simulink model "EV_thermal_charger_2015a_jmaab"  (R2015a)
settings: Solver=ode3  StartTime=0.0  StopTime=1800  FixedStep=sampling_time  RelTol=1e-3
PreLoadFcn:
  | run('init_setting.m')
PostLoadFcn:
  | %set_param(gcs, 'SimulationCommand', 'update');
  | %load('save_param/save_P_Charger', 'P_Charger');
  | %load('save_param/save_T_User_set_temp_degC','T_User_set_temp_degC');
  | %load('save_param/save_ENV_PNT_PTTH_Temp_add_degC','ENV_PNT_PTTH_Temp_add_degC');
  | %load('save_param/save_ENV_PNT_CABIN_Temp_add_degC','ENV_PNT_CABIN_Temp_add_degC');
  | %load('save_param/save_ENV_PNT_PHI_Sunlight_W','ENV_PNT_PHI_Sunlight_W');
  | %load('save_param/save_ENV_PNT_Outside_Temp_ini_degC','ENV_PNT_Outside_Temp_ini_degC');
undefined symbols (not defined in the file or in its folder): BK_PNT_Pow_UL, BK_PNT_ReGene_vel_limit_DN_kmph, BK_PNT_ReGene_vel_limit_UP_kmph, BK_PNT_Tau_brake, Brk_LL, Brk_PGain, Brk_UL, BT_PNT_Hi_C_pol_hi_batt, BT_PNT_Hi_Capa_hi_batt_F, BT_PNT_Hi_ocv_SOC_hi_batt_OCV_V_table, BT_PNT_Hi_ocv_SOC_hi_batt_OCV_V_table_x_SOC, BT_PNT_Hi_R_hi_batt_cell, BT_PNT_Hi_R_pol_hi_batt, BT_PNT_Hi_SOC_MAX_hi_batt, BT_PNT_Hi_SOC_MIN_hi_batt, BT_PNT_Hi_SOC_START_hi_batt, BT_PNT_Lo_Capa_lo_batt_F, BT_PNT_Lo_ocv_SOC_lo_batt_OCV_V_table, BT_PNT_Lo_ocv_SOC_lo_batt_OCV_V_table_x_SOC, BT_PNT_Lo_R_lo_batt_ohm, BT_PNT_Lo_SOC_MAX_lo_batt, BT_PNT_Lo_SOC_MIN_lo_batt, BT_PNT_Lo_SOC_START_lo_batt, BTTH_CNT_P_BT_Heater_W, BTTH_CNT_P_BT_Heater_W_x_BTCells_degC, BTTH_CNT_Voltage_BTFan_V, BTTH_CNT_Voltage_BTFan_V_x_BTCells_degC, BTTH_PNT_BT_Heat_Resi_KpW, BTTH_PNT_BT_Heat_Resi_KpW_x_Wind_m3ps, BTTH_PNT_BT_Heater2BTCells_Heat_Resi_KpW, BTTH_PNT_BT_Heater_Heat_Capa_JpK, BTTH_PNT_BTBlock2BTAir_Heat_Resi_KpW, BTTH_PNT_BTBlock_Heat_Capa_JpK, BTTH_PNT_BTCells2BTBlock_Heat_Resi_KpW, BTTH_PNT_BTCells_Heat_Capa_JpK, BTTH_PNT_v_BTFan_Wind_vel_mps, BTTH_PNT_v_BTFan_Wind_vel_mps_x_V_BTFan, CATH_CNT_P_Aircon_W_LL, CATH_CNT_P_Aircon_W_UL, CATH_CNT_P_Gain_Aircon, CATH_CNT_P_Gain_PTC_Heater, CATH_CNT_P_Gain_SeatHT, CATH_CNT_P_PTC_Heater, CATH_CNT_P_PTC_Heater_W_LL, CATH_CNT_P_PTC_Heater_W_UL, CATH_CNT_P_PTC_Heater_x_T_Outside_temp_degC, CATH_CNT_P_SeatHT_W_LL, CATH_CNT_P_SeatHT_W_UL, CATH_CNT_PGain_Temp_blowout, CATH_CNT_T_Aircon_Indoor_degC, CATH_CNT_T_Aircon_Indoor_degC_x_T_blowout_degC, CATH_CNT_T_PTC_Heater_degC_UL, CATH_CNT_T_SeatHT_Temp_degC, CATH_CNT_T_SeatHT_Temp_degC_x_T_blowout_degC, CATH_CNT_V_HVAC_Fan, CATH_CNT_V_HVAC_Fan_x_T_blowout_degC, CATH_CNT_V_RDFan_V, CATH_CNT_V_RDFan_x_P_Aircon_W, CATH_PNT_Air_Convection_Heat_Resi_KpW, CATH_PNT_Air_Convection_Heat_Resi_x_mps ... (+142)
undefined symbols (not defined in the file): ACC_D_Gain, ACC_I_Gain, ACC_P_Gain
libraries: METI_Lib_vehicle_model x52, simulink x35
(part 3 of 6)

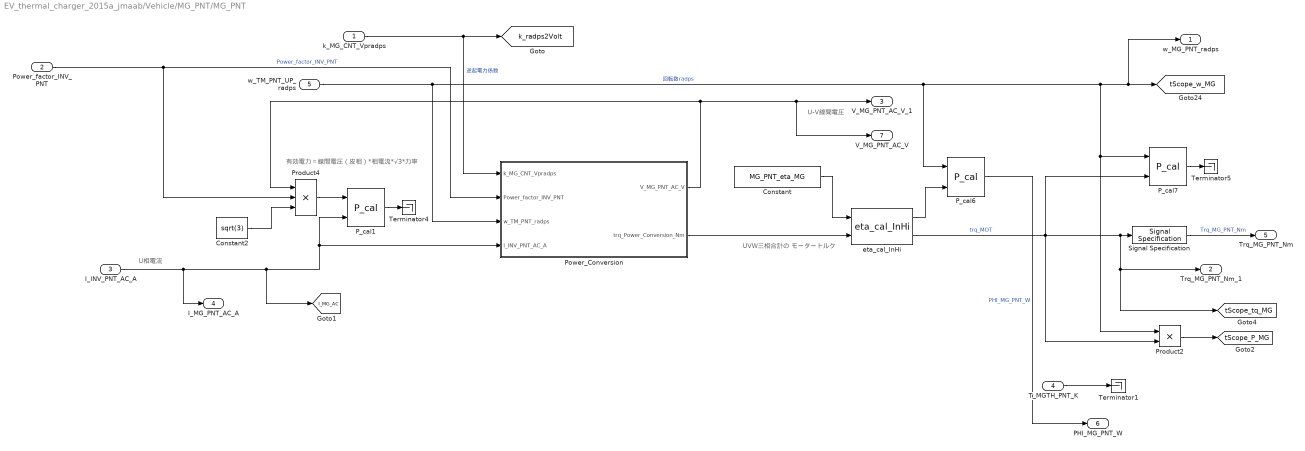
== system EV_thermal_charger_2015a_jmaab/Vehicle/MG_PNT/MG_PNT ==
  note: UVW三相合計の
      | モータートルク
  note: U-V線間電圧
  note: U相電流
  note: 有効電力＝線間電圧（皮相）*相電流*√3*力率
  k_MG_CNT_Vpradps : Inport
  Power_factor_INV_PNT : Inport  Port=2
  "I_INV_PNT_AC_A " : Inport  Port=3
  T_MGTH_PNT_K : Inport  Port=4
  w_TM_PNT_UP_radps : Inport  Port=5
  Constant : Constant  Value=MG_PNT_eta_MG
  Constant2 : Constant  Value=sqrt(3)
  P_cal1 : METI_Lib_vehicle_model/P_cal  Type_energy=電気  Type_output_energy=出力  Power_name=Po_  t_Workspace_Name=MG_PNT_ELEC  P_VariableName=Po_MG_PNT_ELEC  Across_VariableName=V_MG_PNT_ELEC  Throgh_VariableName=I_MG_PNT_ELEC
  P_cal6 : METI_Lib_vehicle_model/P_cal  Type_energy=回転運動  Type_output_energy=損失  Power_name=Pl_  t_Workspace_Name=MG_PNT_FRIC_LOSS  P_VariableName=Pl_MG_PNT_FRIC_LOSS  Across_VariableName=w_MG_PNT_FRIC_LOSS  Throgh_VariableName=tq_MG_PNT_FRIC_LOSS
  P_cal7 : METI_Lib_vehicle_model/P_cal  Type_energy=回転運動  Type_output_energy=出力  Power_name=Po_  t_Workspace_Name=MG_PNT_ROT  P_VariableName=Po_MG_PNT_ROT  Across_VariableName=w_MG_PNT_ROT  Throgh_VariableName=tq_MG_PNT_ROT
  Power_Conversion : Subsystem
  Product2 : Product
  Product4 : Product  Inputs=3
  Signal Specification : SignalSpecification
  Terminator1 : Terminator
  Terminator4 : Terminator
  Terminator5 : Terminator
  eta_cal_InHi : METI_Lib_vehicle_model/eta_cal_InHi  SystemSampleTime=-1
  w_MG_PNT_radps : Outport
  "Trq_MG_PNT_Nm_1 " : Outport  Port=2
  V_MG_PNT_AC_V_1 : Outport  Port=3
  I_MG_PNT_AC_A : Outport  Port=4
  Trq_MG_PNT_Nm : Outport  Port=5
  "PHI_MG_PNT_W " : Outport  Port=6
  "V_MG_PNT_AC_V " : Outport  Port=7
  tag scope: I_MG_AC=global, k_radps2Volt=global, tScope_P_MG=global, tScope_tq_MG=global, tScope_w_MG=global
  wires:
  P_cal1/1 -> Terminator4/1
  P_cal7/1 -> Terminator5/1
  w_TM_PNT_UP_radps/1 -> Power_Conversion/3("w_TM_PNT_radps "), w_MG_PNT_radps/1, [tScope_w_MG], Product2/1, P_cal7/1, P_cal6/1  "回転数radps"
  eta_cal_InHi/2 -> P_cal7/2, Product2/2, [tScope_tq_MG], "Trq_MG_PNT_Nm_1 "/1, Signal Specification/1  "trq_MOT"
  Product2/1 -> [tScope_P_MG]
  P_cal6/1 -> "PHI_MG_PNT_W "/1  "PHI_MG_PNT_W"
  Constant/1 -> eta_cal_InHi/1
  eta_cal_InHi/1 -> P_cal6/2
  k_MG_CNT_Vpradps/1 -> [k_radps2Volt], Power_Conversion/1(k_MG_CNT_Vpradps)  "逆起電力係数"
  Power_Conversion/2("trq_Power_Conversion_Nm ") -> eta_cal_InHi/2
  Power_Conversion/1(V_MG_PNT_AC_V) -> Product4/1, V_MG_PNT_AC_V_1/1, "V_MG_PNT_AC_V "/1
  Product4/1 -> P_cal1/1
  "I_INV_PNT_AC_A "/1 -> [I_MG_AC], P_cal1/2, Power_Conversion/4("I_INV_PNT_AC_A "), I_MG_PNT_AC_A/1
  Power_factor_INV_PNT/1 -> Power_Conversion/2(Power_factor_INV_PNT), Product4/2  "Power_factor_INV_PNT"
  Constant2/1 -> Product4/3
  T_MGTH_PNT_K/1 -> Terminator1/1
  Signal Specification/1 -> Trq_MG_PNT_Nm/1  "Trq_MG_PNT_Nm"

== system EV_thermal_charger_2015a_jmaab/Vehicle/VL_PNT/cal_Hill_Climbing_Resi ==
  note: 登坂抵抗
  In1 : Inport
  Constant2 : Constant  Value=g
  Constant3 : Constant  Value=M
  Gain : Gain  Gain=deg2rad
  Product1 : Product
  Product3 : Product
  Trigonometric Function : Trigonometry
  Out1 : Outport
  wires:
  Trigonometric Function/1 -> Product1/2
  Product1/1 -> Out1/1
  Product3/1 -> Product1/1
  Gain/1 -> Trigonometric Function/1
  Constant2/1 -> Product3/2
  Constant3/1 -> Product3/1
  In1/1 -> Gain/1

== system EV_thermal_charger_2015a_jmaab/Driver/Caliculate_Opeining_Accel/FB/Filter ==
  In1 : Inport
  Gain3 : Gain  Gain=10
  Gain4 : Gain  Gain=0.1
  Rounding Function : Rounding  Operator=round
  Out1 : Outport
  wires:
  Rounding Function/1 -> Gain4/1
  In1/1 -> Gain3/1
  Gain3/1 -> Rounding Function/1
  Gain4/1 -> Out1/1

== system EV_thermal_charger_2015a_jmaab/Driver/Caliculate_Opeining_Accel/FF1/Subsystem ==
  Req_Force : Inport
  Upper_Acc_Force_Input : Inport  Port=2
  Upper_ACC_percent : Inport  Port=3
  Lower_Acc_Force_Input : Inport  Port=4
  Lower_Acc_percent : Inport  Port=5
  Add10 : Sum
  Add11 : Sum  Inputs=+-
  Add8 : Sum  Inputs=+-
  Add9 : Sum  Inputs=+-
  Compare To Zero1 : simulink/Logic and Bit Operations/Compare To Zero  relop=>  OutDataTypeStr=boolean
  Divide_0wari2 : METI_Lib_vehicle_model/Divide_0wari
  Product2 : Product
  Acc_percent_Out : Outport
  threshold_Out : Outport  Port=2
  wires:
  Compare To Zero1/1 -> threshold_Out/1
  Req_Force/1 -> Add9/1
  Lower_Acc_Force_Input/1 -> Add9/2, Add8/2
  Add11/1 -> Product2/2
  Lower_Acc_percent/1 -> Add10/2, Add11/2
  Upper_Acc_Force_Input/1 -> Add8/1
  Product2/1 -> Add10/1
  Add8/1 -> Divide_0wari2/2
  Divide_0wari2/1 -> Product2/1
  Add9/1 -> Compare To Zero1/1, Divide_0wari2/1
  Upper_ACC_percent/1 -> Add11/1
  Add10/1 -> Acc_percent_Out/1

== system EV_thermal_charger_2015a_jmaab/Driver/Caliculate_Opeining_Accel/FF1/Subsystem1 ==
  Req_Force : Inport
  Upper_Acc_Force_Input : Inport  Port=2
  Upper_ACC_percent : Inport  Port=3
  Lower_Acc_Force_Input : Inport  Port=4
  Lower_Acc_percent : Inport  Port=5
  Add10 : Sum
  Add11 : Sum  Inputs=+-
  Add8 : Sum  Inputs=+-
  Add9 : Sum  Inputs=+-
  Compare To Zero1 : simulink/Logic and Bit Operations/Compare To Zero  relop=>  OutDataTypeStr=boolean
  Divide_0wari2 : METI_Lib_vehicle_model/Divide_0wari
  Product2 : Product
  Acc_percent_Out : Outport
  threshold_Out : Outport  Port=2
  wires:
  Compare To Zero1/1 -> threshold_Out/1
  Req_Force/1 -> Add9/1
  Lower_Acc_Force_Input/1 -> Add9/2, Add8/2
  Add11/1 -> Product2/2
  Lower_Acc_percent/1 -> Add10/2, Add11/2
  Upper_Acc_Force_Input/1 -> Add8/1
  Product2/1 -> Add10/1
  Add8/1 -> Divide_0wari2/2
  Divide_0wari2/1 -> Product2/1
  Add9/1 -> Compare To Zero1/1, Divide_0wari2/1
  Upper_ACC_percent/1 -> Add11/1
  Add10/1 -> Acc_percent_Out/1

== system EV_thermal_charger_2015a_jmaab/Driver/Caliculate_Opeining_Accel/FF1/Subsystem2 ==
  Req_Force : Inport
  Upper_Acc_Force_Input : Inport  Port=2
  Upper_ACC_percent : Inport  Port=3
  Lower_Acc_Force_Input : Inport  Port=4
  Lower_Acc_percent : Inport  Port=5
  Add10 : Sum
  Add11 : Sum  Inputs=+-
  Add8 : Sum  Inputs=+-
  Add9 : Sum  Inputs=+-
  Compare To Zero1 : simulink/Logic and Bit Operations/Compare To Zero  relop=>  OutDataTypeStr=boolean
  Divide_0wari2 : METI_Lib_vehicle_model/Divide_0wari
  Product2 : Product
  Acc_percent_Out : Outport
  threshold_Out : Outport  Port=2
  wires:
  Compare To Zero1/1 -> threshold_Out/1
  Req_Force/1 -> Add9/1
  Lower_Acc_Force_Input/1 -> Add9/2, Add8/2
  Add11/1 -> Product2/2
  Lower_Acc_percent/1 -> Add10/2, Add11/2
  Upper_Acc_Force_Input/1 -> Add8/1
  Product2/1 -> Add10/1
  Add8/1 -> Divide_0wari2/2
  Divide_0wari2/1 -> Product2/1
  Add9/1 -> Compare To Zero1/1, Divide_0wari2/1
  Upper_ACC_percent/1 -> Add11/1
  Add10/1 -> Acc_percent_Out/1

== system EV_thermal_charger_2015a_jmaab/Driver/Caliculate_Opeining_Accel/FF1/慣性 ==
  v_tgt : Inport
  Add : Sum
  Constant : Constant  Value=M
  Constant1 : Constant  Value=1/2
  Derivative : Derivative
  Derivative1 : Derivative
  Divide1 : Product  Inputs=***
  Memory : Memory
  F_Inertia : Outport
  wires:
  Divide1/1 -> F_Inertia/1
  v_tgt/1 -> Derivative/1, Memory/1
  Add/1 -> Divide1/2
  Derivative/1 -> Add/1
  Derivative1/1 -> Add/2
  Memory/1 -> Derivative1/1
  Constant1/1 -> Divide1/1
  Constant/1 -> Divide1/3

== system EV_thermal_charger_2015a_jmaab/Driver/Caliculate_Opeining_Accel/FF1/空気抵抗 ==
  v_tgt : Inport
  V_wind : Constant  Value=0
  cal_Air_resi1 : METI_Lib_vehicle_model/vehicle_model/cal_Air_resi  Vel_max=200
  F_air_resi : Outport
  wires:
  cal_Air_resi1/1 -> F_air_resi/1
  V_wind/1 -> cal_Air_resi1/2
  v_tgt/1 -> cal_Air_resi1/1

== system EV_thermal_charger_2015a_jmaab/Driver/Caliculate_Opeining_Accel/FF1/転がり抵抗 ==
  v_tgt : Inport
  cal_roll_resi : METI_Lib_vehicle_model/vehicle_model/cal_roll_resi  Myu_tire=myu  Vehicle_Mass=M  Gravi_acc=g
  F_rollresi : Outport
  wires:
  cal_roll_resi/1 -> F_rollresi/1
  v_tgt/1 -> cal_roll_resi/1

== system EV_thermal_charger_2015a_jmaab/Vehicle/BAT_Hi_PNT/BT_Hi_PNT/Cal_SOC ==
  I_BT_PNT_A : Inport
  Capa_batt : Inport  Port=2
  SOC_st : Inport  Port=3
  SOC_MAX : Inport  Port=4
  SOC_MIN : Inport  Port=5
  Clock : Clock
  Memory : Memory
  Memory1 : Memory
  Saturation Dynamic : simulink/Discontinuities/Saturation Dynamic  OutMin=[]  OutMax=[]  OutDataTypeStr=Inherit: Same as second input  OutDataType=fixdt(1, 16)  OutScaling=2^-10  DoSatur=off
  Subsystem4 : Subsystem  mask{SOC=SOC_LoBat, VariableName=Asec_LoBat}
      mask prompts: SOC "バッテリSOC"; VariableName "バッテリ容量変化量(Asec)"
  Sum : Sum  Inputs=|++
  Sum1 : Sum  Inputs=++|
  Sum2 : Sum  Inputs=+-|
  Sum5 : Sum  Inputs=|+-
  capa_mn : Product  RndMeth=Zero
  capa_mx : Product  RndMeth=Zero
  capa_mx1 : Product  RndMeth=Zero
  capa_st : Product  RndMeth=Zero
  capa_st1 : Product  Inputs=*/  RndMeth=Zero
  h2sec : Gain  Gain=h2sec
  k : Gain  Gain=percent2mujigen
  k1 : Gain  Gain=percent2mujigen
  k2 : Gain  Gain=percent2mujigen
  k3 : Gain  Gain=mujigen2percent
  SOC_out : Outport
  wires:
  Sum5/1 -> capa_mx1/2
  Memory1/1 -> Sum5/2
  Sum/1 -> Saturation Dynamic/2
  Clock/1 -> Sum5/1, Memory1/1
  capa_mx1/1 -> Sum1/1
  k3/1 -> Subsystem4/1(In1), SOC_out/1
  Sum1/1 -> Sum/2
  Memory/1 -> Sum1/2
  k2/1 -> capa_st/2
  k1/1 -> capa_mn/2
  k/1 -> capa_mx/2
  capa_st/1 -> Sum2/2, Sum/1
  Saturation Dynamic/1 -> Sum2/1, capa_st1/1
  capa_mx/1 -> Saturation Dynamic/1
  capa_mn/1 -> Saturation Dynamic/3
  capa_st1/1 -> k3/1
  h2sec/1 -> capa_mn/1, capa_st1/2, capa_st/1, capa_mx/1
  SOC_MIN/1 -> k1/1
  SOC_MAX/1 -> k/1
  SOC_st/1 -> k2/1
  Capa_batt/1 -> h2sec/1
  I_BT_PNT_A/1 -> capa_mx1/1
  Sum2/1 -> Memory/1, Subsystem4/2(In2)

== system EV_thermal_charger_2015a_jmaab/Vehicle/BAT_Hi_PNT/BT_Hi_PNT/Subsystem ==
  I_BT_PNT_A : Inport
  Add : Sum
  Divide : Product
  Resistivity : Constant  Value=BT_PNT_Hi_R_hi_batt_cell
  Transfer Fcn : TransferFcn  Numerator=[BT_PNT_Hi_R_pol_hi_batt]  Denominator=[BT_PNT_Hi_R_pol_hi_batt*BT_PNT_Hi_C_pol_hi_batt 1]
  V_BT_PNT_V : Outport
  wires:
  Resistivity/1 -> Divide/2
  I_BT_PNT_A/1 -> Transfer Fcn/1, Divide/1
  Divide/1 -> Add/1
  Transfer Fcn/1 -> Add/2
  Add/1 -> V_BT_PNT_V/1

== system EV_thermal_charger_2015a_jmaab/Vehicle/BTTH/BTTH_PNT/BB_PNT ==
  note: バッテリ筐体の
      | 熱容量
  ini_T_Environment_Outside_degC : Inport
  T_ATM_PNT_BB_K : Inport  Port=2
  PHI_BTBlock1_W : Inport  Port=3
  BTBlock_Heat_Capacity : Subsystem
  BT_Block2Air_Heat_Resistance : Subsystem
  T_BTBlock1_K : Outport
  PHI_BB_PNT_ATM_W : Outport  Port=2
  T_BTBlock2_K : Outport  Port=3
  wires:
  ini_T_Environment_Outside_degC/1 -> BTBlock_Heat_Capacity/1(ini_T_Environment_Outside_degC)
  BTBlock_Heat_Capacity/1(T_BTBlock1_K) -> T_BTBlock1_K/1
  PHI_BTBlock1_W/1 -> BTBlock_Heat_Capacity/2(PHI_BTBlock1_W)
  BT_Block2Air_Heat_Resistance/1(PHI_BT2AIR_Resi1_W) -> PHI_BB_PNT_ATM_W/1  "PHI_BB_PNT_ATM_W"
  BT_Block2Air_Heat_Resistance/2(PHI_BTBlock_Resi2_W) -> BTBlock_Heat_Capacity/3(PHI_BTBlock2_W)
  T_ATM_PNT_BB_K/1 -> BT_Block2Air_Heat_Resistance/1(T_ATM_PNT_BB_K)
  BTBlock_Heat_Capacity/2(T_BTBlock2_K) -> T_BTBlock2_K/1, BT_Block2Air_Heat_Resistance/2(T_BTBlock_Resi2_K)

== system EV_thermal_charger_2015a_jmaab/Vehicle/BTTH/BTTH_PNT/BC_PNT ==
  note: バッテリセルの
      | 熱容量
  PHI_BTCells4_W : Inport
  T_BTBlock_Resi1_K : Inport  Port=2
  ini_T_Environment_Outside_degC : Inport  Port=3
  PHI_BTCells2_W : Inport  Port=4
  PHI_BT_HI_PNT_W : Inport  Port=5
  BTCells_Heat_Capacity : Subsystem
  BT_Cells2BTBlock_Heat_Resistance : Subsystem
  T_BTCells4_K : Outport
  PHI_BTBlock_Resi1_W : Outport  Port=2
  T_BC_PNT_K : Outport  Port=3
  T_BTCCell_K : Outport  Port=4
  T_BTCells2_K : Outport  Port=5
  wires:
  BTCells_Heat_Capacity/2(T_BTCells2_K) -> T_BTCells2_K/1
  PHI_BTCells2_W/1 -> BTCells_Heat_Capacity/3(PHI_BTCells2_W)
  ini_T_Environment_Outside_degC/1 -> BTCells_Heat_Capacity/1(ini_T_Environment_Outside_degC)
  PHI_BT_HI_PNT_W/1 -> BTCells_Heat_Capacity/2(PHI_BTCells1_W)
  PHI_BTCells4_W/1 -> BTCells_Heat_Capacity/5(PHI_BTCells4_W)
  BT_Cells2BTBlock_Heat_Resistance/2(PHI_BTCells_Resi2_W) -> BTCells_Heat_Capacity/4(PHI_BTCells3_W)
  BT_Cells2BTBlock_Heat_Resistance/1(PHI_BTBlock_Resi1_W) -> PHI_BTBlock_Resi1_W/1
  BTCells_Heat_Capacity/1(T_BTCells1_K) -> T_BC_PNT_K/1  "T_BC_PNT_K"
  T_BTBlock_Resi1_K/1 -> BT_Cells2BTBlock_Heat_Resistance/1(T_BTBlock_Resi1_K)
  BTCells_Heat_Capacity/4(T_BTCells4_K) -> T_BTCells4_K/1
  BTCells_Heat_Capacity/3(T_BTCells3_K) -> T_BTCCell_K/1, BT_Cells2BTBlock_Heat_Resistance/2(T_BTCells_Resi2_K)

== system EV_thermal_charger_2015a_jmaab/Vehicle/BTTH/BTTH_PNT/BF_PNT ==
  V_BTTH_CNT_BTFan_V : Inport
  T_ATM_PNT_BF_K : Inport  Port=2
  T_BT_Fan_Resi2_K : Inport  Port=3
  BTFan_Heat_Resistance : Subsystem
  BT_Fan_Heat_Resi_Calc : Subsystem
  PHI_BT_Fan_Resi2_W : Outport
  PHI_BF_PNT_ATM_W : Outport  Port=2
  wires:
  BTFan_Heat_Resistance/2(PHI_BT_Fan_Resi2_W) -> PHI_BT_Fan_Resi2_W/1  "PHI_BT_Fan_Resi2_W"
  T_BT_Fan_Resi2_K/1 -> BTFan_Heat_Resistance/3(T_BT_Fan_Resi2_K)
  T_ATM_PNT_BF_K/1 -> BTFan_Heat_Resistance/2(T_ATM_PNT_BF_K)
  BTFan_Heat_Resistance/1(PHI_BT_Fan_Resi1_W) -> PHI_BF_PNT_ATM_W/1  "PHI_BF_PNT_ATM_W"
  V_BTTH_CNT_BTFan_V/1 -> BT_Fan_Heat_Resi_Calc/1(BTTH_PNT_Voltage_BTFan_V)
  BT_Fan_Heat_Resi_Calc/1("BTTH_PNT_BTFan_Heat_Resi_KpW ") -> BTFan_Heat_Resistance/1("BTTH_PNT_BTFan_Heat_Resi_KpW ")

== system EV_thermal_charger_2015a_jmaab/Vehicle/BTTH/BTTH_PNT/BH_PNT ==
  note: バッテリヒータの
      | 熱容量
  ini_T_Environment_Outside_degC : Inport
  tgt_P_BTTH_CNT_BTHeater_W : Inport  Port=2
  V_BT_Lo_PNT_V : Inport  Port=3
  T_BTCells_Resi1_K : Inport  Port=4
  BT_Heater : Subsystem
  BT_Heater2BTCells_Heat_Resistance : Subsystem
  BT_Heater_Heat_Capacity : Subsystem
  Gain : Gain  Gain=-1
  P_cal : METI_Lib_vehicle_model/P_cal  Type_energy=電気  Type_output_energy=損失  Power_name=Pl_  t_Workspace_Name=BT_Heater_Elec  P_VariableName=Pl_BT_Heater_Elec  Across_VariableName=V_BT_Heater_Elec  Throgh_VariableName=I_BT_Heater_Elec
  Terminator : Terminator
  PHI_BTCells_Resi1_W : Outport
  I_BTTH_PNT_A : Outport  Port=2
  wires:
  ini_T_Environment_Outside_degC/1 -> BT_Heater_Heat_Capacity/1(PHI_BTCells_Resi1_W)
  BT_Heater2BTCells_Heat_Resistance/1(PHI_BTCells_Resi1_W) -> PHI_BTCells_Resi1_W/1
  BT_Heater2BTCells_Heat_Resistance/2(PHI_BT_Heater_Resi2_W) -> BT_Heater_Heat_Capacity/3(PHI_BT_Heater2_W)
  BT_Heater/1(PHI_BT_Heater_W) -> BT_Heater_Heat_Capacity/2(PHI_BT_Heater1_W)
  V_BT_Lo_PNT_V/1 -> P_cal/1, BT_Heater/3(V_BT_Lo_PNT_V)
  Gain/1 -> P_cal/2
  BT_Heater/2(I_BT_Heater_A) -> I_BTTH_PNT_A/1, Gain/1  "I_BTTH_PNT_A"
  tgt_P_BTTH_CNT_BTHeater_W/1 -> BT_Heater/2(tgt_P_BTTH_CNT_BTHeater_W)
  P_cal/1 -> Terminator/1
  BT_Heater_Heat_Capacity/1(T_BT_Heater1_K) -> BT_Heater/1(T_BT_Heater_K)
  BT_Heater_Heat_Capacity/2(T_BT_Heater2_K) -> BT_Heater2BTCells_Heat_Resistance/2(T_BT_Heater_Resi2_K)
  T_BTCells_Resi1_K/1 -> BT_Heater2BTCells_Heat_Resistance/1(T_BTCells_Resi1_K)

== system EV_thermal_charger_2015a_jmaab/Vehicle/BTTH/BTTH_PNT/K->degC ==
  K : Inport
  Constant2 : Constant  Value=K2degC
  Sum : Sum  Inputs=++|
  degC : Outport
  wires:
  K/1 -> Sum/2
  Constant2/1 -> Sum/1
  Sum/1 -> degC/1

== system EV_thermal_charger_2015a_jmaab/Vehicle/BTTH/BTTH_PNT/K->degC1 ==
  K : Inport
  Constant2 : Constant  Value=K2degC
  Sum : Sum  Inputs=++|
  degC : Outport
  wires:
  K/1 -> Sum/2
  Constant2/1 -> Sum/1
  Sum/1 -> degC/1

== system EV_thermal_charger_2015a_jmaab/Vehicle/BT_Lo_PNT/BT_Lo_PNT/Cal_SOC ==
  I_Lo_BT_PNT_A : Inport
  Capa_batt : Inport  Port=2
  SOC_st : Inport  Port=3
  SOC_MAX : Inport  Port=4
  SOC_MIN : Inport  Port=5
  Clock : Clock
  Memory : Memory
  Memory1 : Memory
  Saturation Dynamic : simulink/Discontinuities/Saturation Dynamic  OutMin=[]  OutMax=[]  OutDataTypeStr=Inherit: Same as second input  OutDataType=fixdt(1, 16)  OutScaling=2^-10  DoSatur=off
  Sum : Sum  Inputs=|++
  Sum1 : Sum  Inputs=++|
  Sum2 : Sum  Inputs=+-|
  Sum5 : Sum  Inputs=|+-
  capa_mn : Product  RndMeth=Zero
  capa_mx : Product  RndMeth=Zero
  capa_mx1 : Product  RndMeth=Zero
  capa_st : Product  RndMeth=Zero
  capa_st1 : Product  Inputs=*/  RndMeth=Zero
  h2sec : Gain  Gain=h2sec
  k : Gain  Gain=percent2mujigen
  k1 : Gain  Gain=percent2mujigen
  k2 : Gain  Gain=percent2mujigen
  k3 : Gain  Gain=mujigen2percent
  SOC_out : Outport
  wires:
  Sum5/1 -> capa_mx1/2
  Memory1/1 -> Sum5/2
  Sum/1 -> Saturation Dynamic/2
  Clock/1 -> Sum5/1, Memory1/1
  capa_mx1/1 -> Sum1/1
  k3/1 -> SOC_out/1
  Sum1/1 -> Sum/2
  Memory/1 -> Sum1/2
  k2/1 -> capa_st/2
  k1/1 -> capa_mn/2
  k/1 -> capa_mx/2
  capa_st/1 -> Sum2/2, Sum/1
  Saturation Dynamic/1 -> Sum2/1, capa_st1/1
  capa_mx/1 -> Saturation Dynamic/1
  capa_mn/1 -> Saturation Dynamic/3
  capa_st1/1 -> k3/1
  h2sec/1 -> capa_mn/1, capa_st1/2, capa_st/1, capa_mx/1
  SOC_MIN/1 -> k1/1
  SOC_MAX/1 -> k/1
  SOC_st/1 -> k2/1
  Capa_batt/1 -> h2sec/1
  I_Lo_BT_PNT_A/1 -> capa_mx1/1
  Sum2/1 -> Memory/1

== system EV_thermal_charger_2015a_jmaab/Vehicle/BT_Lo_PNT/BT_Lo_PNT/Subsystem ==
  I_BT_PNT_Lo_A : Inport
  Divide : Product
  Resistivity : Constant  Value=BT_PNT_Lo_R_lo_batt_ohm
  V_BT_PNT_Lo_V : Outport
  wires:
  Resistivity/1 -> Divide/2
  I_BT_PNT_Lo_A/1 -> Divide/1
  Divide/1 -> V_BT_PNT_Lo_V/1

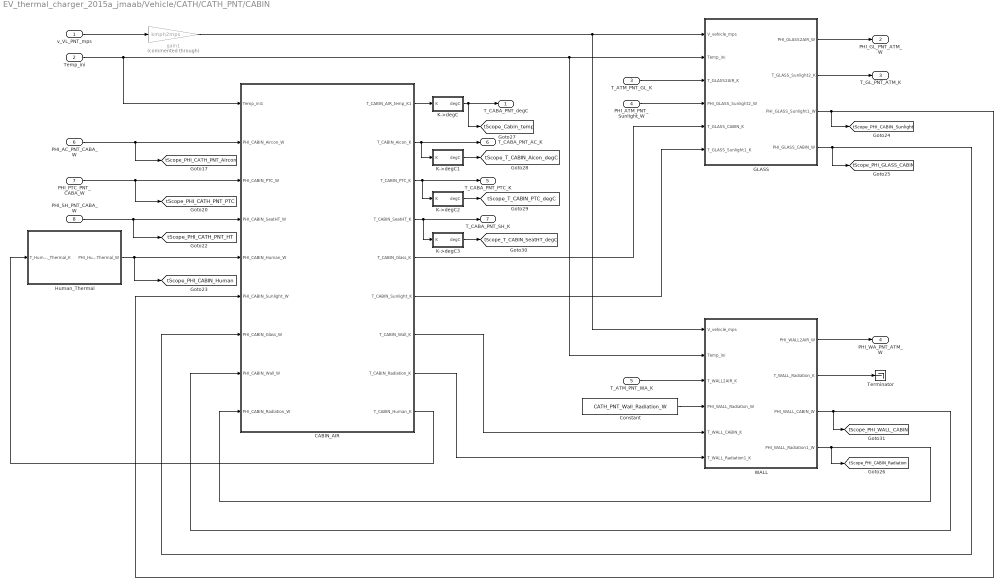
== system EV_thermal_charger_2015a_jmaab/Vehicle/CATH/CATH_PNT/CABIN ==
  v_VL_PNT_mps : Inport
  Temp_ini : Inport  Port=2
  T_ATM_PNT_GL_K : Inport  Port=3
  PHI_ATM_PNT_Sunlight_W : Inport  Port=4
  T_ATM_PNT_WA_K : Inport  Port=5
  PHI_AC_PNT_CABA_W : Inport  Port=6
  PHI_PTC_PNT_CABA_W : Inport  Port=7
  PHI_SH_PNT_CABA_W : Inport  Port=8
  CABIN_AIR : Subsystem
  Constant : Constant  Value=CATH_PNT_Wall_Radiation_W
  GLASS : Subsystem
  Human_Thermal : Subsystem
  K->degC : Subsystem
  K->degC1 : Subsystem
  K->degC2 : Subsystem
  K->degC3 : Subsystem
  Terminator : Terminator
  WALL : Subsystem
  gain1 : Gain  Commented=through  Gain=kmph2mps
  T_CABA_PNT_degC : Outport
  PHI_GL_PNT_ATM_W : Outport  Port=2
  T_GL_PNT_ATM_K : Outport  Port=3
  PHI_WA_PNT_ATM_W : Outport  Port=4
  T_CABA_PNT_PTC_K : Outport  Port=5
  T_CABA_PNT_AC_K : Outport  Port=6
  T_CABA_PNT_SH_K : Outport  Port=7
  tag scope: tScope_Cabin_temp=global, tScope_PHI_CABIN_Human=global, tScope_PHI_CABIN_Radiation=global, tScope_PHI_CABIN_Sunlight=global, tScope_PHI_CATH_PNT_Aircon=global, tScope_PHI_CATH_PNT_HT=global, tScope_PHI_CATH_PNT_PTC=global, tScope_PHI_GLASS_CABIN=global, tScope_PHI_WALL_CABIN=global, tScope_T_CABIN_Aicon_degC=global, tScope_T_CABIN_PTC_degC=global, tScope_T_CABIN_SeatHT_degC=global
  wires:
  CABIN_AIR/6(T_CABIN_Sunlight_K) -> GLASS/6(T_GLASS_Sunlight1_K)
  T_ATM_PNT_GL_K/1 -> GLASS/3(T_GLASS2AIR_K)
  GLASS/1(PHI_GLASS2AIR_W) -> PHI_GL_PNT_ATM_W/1
  CABIN_AIR/8(T_CABIN_Radiation_K) -> WALL/6(T_WALL_Radiation1_K)
  WALL/1(PHI_WALL2AIR_W) -> PHI_WA_PNT_ATM_W/1
  T_ATM_PNT_WA_K/1 -> WALL/3(T_WALL2AIR_K)
  CABIN_AIR/9(T_CABIN_Human_K) -> Human_Thermal/1(T_Human_Thermal_K)
  GLASS/2(T_GLASS_Sunlight2_K) -> T_GL_PNT_ATM_K/1
  PHI_ATM_PNT_Sunlight_W/1 -> GLASS/4(PHI_GLASS_Sunlight2_W)
  CABIN_AIR/1(T_CABIN_AIR_temp_K1) -> K->degC/1(K)
  K->degC/1(degC) -> T_CABA_PNT_degC/1, [tScope_Cabin_temp]
  Temp_ini/1 -> GLASS/2(Temp_ini), WALL/2(Temp_ini), CABIN_AIR/1(Temp_ini1)
  CABIN_AIR/5(T_CABIN_Glass_K) -> GLASS/5(T_GLASS_CABIN_K)
  CABIN_AIR/7(T_CABIN_Wall_K) -> WALL/5(T_WALL_CABIN_K)
  v_VL_PNT_mps/1 -> gain1/1
  Constant/1 -> WALL/4(PHI_WALL_Radiation_W)
  WALL/2(T_WALL_Radiation_K) -> Terminator/1
  gain1/1 -> GLASS/1(V_vehicle_mps), WALL/1(V_vehicle_mps)
  Human_Thermal/1(PHI_Human_Thermal_W) -> [tScope_PHI_CABIN_Human], CABIN_AIR/5(PHI_CABIN_Human_W)
  K->degC1/1(degC) -> [tScope_T_CABIN_Aicon_degC]
  K->degC2/1(degC) -> [tScope_T_CABIN_PTC_degC]
  K->degC3/1(degC) -> [tScope_T_CABIN_SeatHT_degC]
  PHI_AC_PNT_CABA_W/1 -> CABIN_AIR/2(PHI_CABIN_Aircon_W), [tScope_PHI_CATH_PNT_Aircon]
  PHI_PTC_PNT_CABA_W/1 -> [tScope_PHI_CATH_PNT_PTC], CABIN_AIR/3(PHI_CABIN_PTC_W)
  PHI_SH_PNT_CABA_W/1 -> [tScope_PHI_CATH_PNT_HT], CABIN_AIR/4(PHI_CABIN_SeatHT_W)
  CABIN_AIR/2(T_CABIN_Aicon_K) -> T_CABA_PNT_AC_K/1, K->degC1/1(K)
  CABIN_AIR/3(T_CABIN_PTC_K) -> T_CABA_PNT_PTC_K/1, K->degC2/1(K)
  CABIN_AIR/4(T_CABIN_SeatHT_K) -> T_CABA_PNT_SH_K/1, K->degC3/1(K)
  GLASS/3(PHI_GLASS_Sunlight1_W) -> CABIN_AIR/6(PHI_CABIN_Sunlight_W), [tScope_PHI_CABIN_Sunlight]
  WALL/4(PHI_WALL_Radiation1_W) -> [tScope_PHI_CABIN_Radiation], CABIN_AIR/9(PHI_CABIN_Radiation_W)
  GLASS/4(PHI_GLASS_CABIN_W) -> [tScope_PHI_GLASS_CABIN], CABIN_AIR/7(PHI_CABIN_Glass_W)
  WALL/3(PHI_WALL_CABIN_W) -> [tScope_PHI_WALL_CABIN], CABIN_AIR/8(PHI_CABIN_Wall_W)

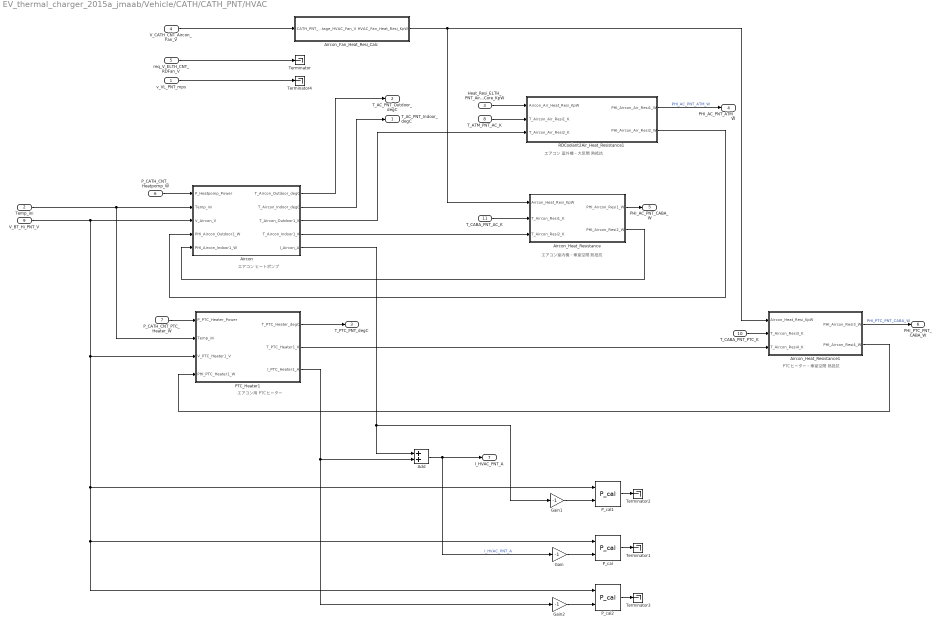
== system EV_thermal_charger_2015a_jmaab/Vehicle/CATH/CATH_PNT/HVAC ==
  note: エアコン用
      | PTCヒーター
  note: エアコン
      | ヒートポンプ
  note: エアコン 室外機～大気間
      | 熱抵抗
  note: エアコン室内機～車室空間
      | 熱抵抗
  note: PTCヒーター～車室空間
      | 熱抵抗
  v_VL_PNT_mps : Inport
  Temp_ini : Inport  Port=2
  Heat_Resi_ELTH_PNT_AirconCore_KpW : Inport  Port=3
  V_CATH_CNT_Aircon_Fan_V : Inport  Port=4
  req_V_ELTH_CNT_RDFan_V : Inport  Port=5
  P_CATH_CNT_Heatpomp_W : Inport  Port=6
  P_CATH_CNT_PTC_Heater_W : Inport  Port=7
  T_ATM_PNT_AC_K : Inport  Port=8
  V_BT_Hi_PNT_V : Inport  Port=9
  T_CABA_PNT_PTC_K : Inport  Port=10
  T_CABA_PNT_AC_K : Inport  Port=11
  Add : Sum
  Aircon : Subsystem
  Aircon_Fan_Heat_Resi_Calc : Subsystem
  Aircon_Heat_Resistance : Subsystem
  Aircon_Heat_Resistance1 : Subsystem
  Gain : Gain  Gain=-1
  Gain1 : Gain  Gain=-1
  Gain2 : Gain  Gain=-1
  PTC_Heater1 : Subsystem
  P_cal : METI_Lib_vehicle_model/P_cal  Type_energy=電気  Type_output_energy=損失  Power_name=Pl_  t_Workspace_Name=EL_HVAC  P_VariableName=Pl_EL_HVAC  Across_VariableName=V_EL_HVAC  Throgh_VariableName=I_EL_HVAC
  P_cal1 : METI_Lib_vehicle_model/P_cal  Type_energy=電気  Type_output_energy=損失  Power_name=Pl_  t_Workspace_Name=EL_Aircon_Comp  P_VariableName=Pl_EL_Aircon_Comp  Across_VariableName=V_EL_Aircon_Comp  Throgh_VariableName=I_EL_Aircon_Comp
  P_cal2 : METI_Lib_vehicle_model/P_cal  Type_energy=電気  Type_output_energy=損失  Power_name=Pl_  t_Workspace_Name=EL_HVAC_PTC  P_VariableName=Pl_EL_HVAC_PTC  Across_VariableName=V_EL_HVAC_PTC  Throgh_VariableName=I_EL_HVAC_PTC
  RDCoolant2Air_Heat_Resistance1 : Subsystem
  Terminator{,1..4} (5 alike) : Terminator
  T_AC_PNT_Indoor_degC : Outport
  T_AC_PNT_Outdoor_degC : Outport  Port=2
  T_PTC_PNT_degC : Outport  Port=3
  PHI_AC_PNT_ATM_W : Outport  Port=4
  PHI_AC_PNT_CABA_W : Outport  Port=5
  PHI_PTC_PNT_CABA_W : Outport  Port=6
  I_HVAC_PNT_A : Outport  Port=7
  wires:
  T_ATM_PNT_AC_K/1 -> RDCoolant2Air_Heat_Resistance1/2(T_Aircon_Air_Resi1_K)
  T_CABA_PNT_AC_K/1 -> Aircon_Heat_Resistance/2(T_Aircon_Resi1_K)
  Add/1 -> I_HVAC_PNT_A/1, Gain/1  "I_HVAC_PNT_A"
  RDCoolant2Air_Heat_Resistance1/1(PHI_Aircon_Air_Resi1_W) -> PHI_AC_PNT_ATM_W/1  "PHI_AC_PNT_ATM_W"
  Aircon_Heat_Resistance/1(PHI_Aircon_Resi1_W) -> PHI_AC_PNT_CABA_W/1
  Aircon_Heat_Resistance1/1(PHI_Aircon_Resi3_W) -> PHI_PTC_PNT_CABA_W/1  "PHI_PTC_PNT_CABA_W"
  T_CABA_PNT_PTC_K/1 -> Aircon_Heat_Resistance1/2(T_Aircon_Resi3_K)
  Aircon/3(T_Aircon_Outdoor1_K) -> RDCoolant2Air_Heat_Resistance1/3(T_Aircon_Air_Resi2_K)
  req_V_ELTH_CNT_RDFan_V/1 -> Terminator/1
  Heat_Resi_ELTH_PNT_AirconCore_KpW/1 -> RDCoolant2Air_Heat_Resistance1/1("Aircon_Air_Heat_Resi_KpW ")
  RDCoolant2Air_Heat_Resistance1/2(PHI_Aircon_Air_Resi2_W) -> Aircon/4(PHI_Aircon_Outdoor1_W)
  v_VL_PNT_mps/1 -> Terminator4/1
  Aircon_Heat_Resistance/2(PHI_Aircon_Resi2_W) -> Aircon/5(PHI_Aircon_Indoor1_W)
  P_CATH_CNT_PTC_Heater_W/1 -> PTC_Heater1/1(P_PTC_Heater_Power)
  PTC_Heater1/3(I_PTC_Heater1_A) -> Gain2/1, Add/2
  P_CATH_CNT_Heatpomp_W/1 -> Aircon/1(P_Heatpomp_Power)
  Temp_ini/1 -> Aircon/2(Temp_ini), PTC_Heater1/2(Temp_ini)
  Aircon/5(I_Aircon_A) -> Gain1/1, Add/1
  Aircon_Fan_Heat_Resi_Calc/1("HVAC_Fan_Heat_Resi_KpW ") -> Aircon_Heat_Resistance/1("Aircon_Heat_Resi_KpW "), Aircon_Heat_Resistance1/1("Aircon_Heat_Resi_KpW ")
  V_CATH_CNT_Aircon_Fan_V/1 -> Aircon_Fan_Heat_Resi_Calc/1(CATH_PNT_Voltage_HVAC_Fan_V)
  Aircon/2(T_Aircon_Indoor_degC) -> T_AC_PNT_Indoor_degC/1
  PTC_Heater1/1(T_PTC_Heater_degC) -> T_PTC_PNT_degC/1
  PTC_Heater1/2(T_PTC_Heater1_K) -> Aircon_Heat_Resistance1/3(T_Aircon_Resi4_K)
  Aircon_Heat_Resistance1/2(PHI_Aircon_Resi4_W) -> PTC_Heater1/4(PHI_PTC_Heater1_W)
  Aircon/4(T_Aircon_Indoor1_K) -> Aircon_Heat_Resistance/3(T_Aircon_Resi2_K)
  Aircon/1(T_Aircon_Outdoor_degC) -> T_AC_PNT_Outdoor_degC/1
  P_cal/1 -> Terminator1/1
  Gain/1 -> P_cal/2
  P_cal1/1 -> Terminator2/1
  Gain1/1 -> P_cal1/2
  P_cal2/1 -> Terminator3/1
  V_BT_Hi_PNT_V/1 -> P_cal2/1, P_cal/1, P_cal1/1, PTC_Heater1/3(V_PTC_Heater1_V), Aircon/3(V_Aircon_V)
  Gain2/1 -> P_cal2/2

== system EV_thermal_charger_2015a_jmaab/Vehicle/CATH/CATH_PNT/Seat_Heater ==
  Temp_ini : Inport
  P_CATH_CNT_SeatHT_W : Inport  Port=2
  V_BT_Lo_PNT_V : Inport  Port=3
  T_CABA_PNT_SH_K : Inport  Port=4
  Gain : Gain  Gain=-1
  K->degC : Subsystem
  P_cal : METI_Lib_vehicle_model/P_cal  Type_energy=電気  Type_output_energy=損失  Power_name=Pl_  t_Workspace_Name=EL_Seat_Heater  P_VariableName=Pl_EL_Seat_Heater  Across_VariableName=V_EL_Seat_Heater  Throgh_VariableName=I_EL_Seat_Heater
  SeatHT_Heat_Capacity : Subsystem
  Seat_HT : Subsystem
  Seat_Heater_Heat_Resistance : Subsystem
  Terminator1 : Terminator
  PHI_SH_PNT_CABA_W : Outport
  T_SeatHT_Temp_degC : Outport  Port=2
  I_Seat_HT_A : Outport  Port=3
  wires:
  SeatHT_Heat_Capacity/2(T_SeatHT1_K) -> Seat_HT/3(T_Seat_HT_K)
  Seat_Heater_Heat_Resistance/2(PHI_SeatHT_Resi2_W) -> SeatHT_Heat_Capacity/3(PHI_SeatHT2_W)
  SeatHT_Heat_Capacity/1(T_SeatHT2_K) -> Seat_Heater_Heat_Resistance/1(T_SeatHT_Resi2_K), K->degC/1(K)
  Temp_ini/1 -> SeatHT_Heat_Capacity/1(Temp_ini)
  T_CABA_PNT_SH_K/1 -> Seat_Heater_Heat_Resistance/2(T_SeatHT_Resi1_K)
  Seat_Heater_Heat_Resistance/1(PHI_SeatHT_Resi1_W) -> PHI_SH_PNT_CABA_W/1  "PHI_SH_PNT_CABA_W"
  K->degC/1(degC) -> T_SeatHT_Temp_degC/1  "T_SeatHT_Temp_degC"
  P_CATH_CNT_SeatHT_W/1 -> Seat_HT/1(P_Seat_Heater_Power)
  Seat_HT/2(I_Seat_HT_A) -> I_Seat_HT_A/1, Gain/1
  P_cal/1 -> Terminator1/1
  Gain/1 -> P_cal/2
  V_BT_Lo_PNT_V/1 -> Seat_HT/2(V_Seat_HT_V), P_cal/1
  Seat_HT/1(PHI_Seat_HT_W) -> SeatHT_Heat_Capacity/2(PHI_SeatHT1_W)

== system EV_thermal_charger_2015a_jmaab/Vehicle/CNT/BK_CNT/BK_CNT ==
  note: ～回生協調ブレーキ時～
      | 実際に出力できている回生ブレーキ力を受け取り
      | メカブレーキ負担分から減算することで
      | 車両としてのブレーキ力が
      | ドライバ操作通りになるようにする
  open_brake_Driver_per : Inport
  F_VCU_CNT_re_brake_N : Inport  Port=2
  Add : Sum
  Constant : Constant  Value=0
  Constant1 : Constant  Value=-inf
  Constant2 : Constant  Value=BK_PNT_Pow_UL
  Constant3 : Constant  Value=0
  Constant4 : Constant  Value=inf
  Constant5 : Constant  Value=BK_PNT_Pow_UL
  Divide : Product  Inputs=*/
  Product1 : Product
  Saturation Dynamic : simulink/Discontinuities/Saturation Dynamic  OutMin=[]  OutMax=[]  OutDataTypeStr=Inherit: Same as second input  OutDataType=fixdt(1, 16)  OutScaling=2^-10  DoSatur=off
  Saturation Dynamic1 : simulink/Discontinuities/Saturation Dynamic  OutMin=[]  OutMax=[]  OutDataTypeStr=Inherit: Same as second input  OutDataType=fixdt(1, 16)  OutScaling=2^-10  DoSatur=off
  per2F : Gain  Gain=1/100
  per2F1 : Gain  Gain=100
  open_brake_BK_CNT_per : Outport
  wires:
  F_VCU_CNT_re_brake_N/1 -> Saturation Dynamic/2  "F_VCU_CNT_re_brake_N"
  open_brake_Driver_per/1 -> per2F/1  "open_brake_Driver_per"
  Add/1 -> Saturation Dynamic1/2
  per2F/1 -> Product1/1
  Constant2/1 -> Product1/2
  Saturation Dynamic1/1 -> Divide/1
  Constant/1 -> Saturation Dynamic/1
  Constant1/1 -> Saturation Dynamic/3
  Constant3/1 -> Saturation Dynamic1/3
  Constant4/1 -> Saturation Dynamic1/1
  Product1/1 -> Add/1
  Saturation Dynamic/1 -> Add/2
  Constant5/1 -> Divide/2
  Divide/1 -> per2F1/1
  per2F1/1 -> open_brake_BK_CNT_per/1

== system EV_thermal_charger_2015a_jmaab/Vehicle/CNT/BTTH_CNT/BTTH_CNT ==
  T_BC_PNT_degC : Inport
  1-D Lookup Table : Lookup_n-D  NumberOfTableDimensions=1  BreakpointsForDimension1=BTTH_CNT_P_BT_Heater_W_x_BTCells_degC  Table=BTTH_CNT_P_BT_Heater_W  InternalRulePriority=Speed  RndMeth=Simplest  InputSameDT=on
  1-D Lookup Table1 : Lookup_n-D  NumberOfTableDimensions=1  BreakpointsForDimension1=BTTH_CNT_Voltage_BTFan_V_x_BTCells_degC  Table=BTTH_CNT_Voltage_BTFan_V  InternalRulePriority=Speed  RndMeth=Simplest  InputSameDT=on
  tgt_P_BTTH_CNT_BTHeater_W : Outport
  V_BTTH_CNT_BTFan_V : Outport  Port=2
  wires:
  1-D Lookup Table/1 -> tgt_P_BTTH_CNT_BTHeater_W/1  "tgt_P_BTTH_CNT_BTHeater_W"
  1-D Lookup Table1/1 -> V_BTTH_CNT_BTFan_V/1  "V_BTTH_CNT_BTFan_V"
  T_BC_PNT_degC/1 -> 1-D Lookup Table1/1, 1-D Lookup Table/1  "T_BC_PNT_degC"

== system EV_thermal_charger_2015a_jmaab/Vehicle/CNT/CATH_CNT/CATH_CNT ==
  note: ヒートポンプパワー＞0 → 車室への熱量＞0 ＝暖房
      |
      | ヒートポンプ パワー＜0 → 車室への熱量＜0 ＝冷房
  tSetting_P_Charger : Inport
  tSetting_T_User_set_temp_degC : Inport  Port=2
  T_ATM_PNT_Outside_degC : Inport  Port=3
  T_CABA_PNT_degC : Inport  Port=4
  T_SH_PNT_degC : Inport  Port=5
  T_AC_PNT_Indoor_degC : Inport  Port=6
  T_PTC_PNT_degC : Inport  Port=7
  v_VL_PNT_kmph : Inport  Port=8
  Calc_Temp_Blowout : Subsystem
  P_Heatpomp_Power_tgt_calc : Subsystem
  P_PTC_Heater_tgt_calc : Subsystem
  Subsystem1 : Subsystem
  T_SeatHT_Temp_tgt_calc : Subsystem
  Terminator1 : Terminator
  V_HVAC_Fan_calc : Subsystem
  V_CATH_CNT_Aircon_Fan_V : Outport
  P_CATH_CNT_Heatpomp_W : Outport  Port=2
  req_V_CATH_CNT_RDFan_V : Outport  Port=3
  P_CATH_CNT_PTC_Heater_W : Outport  Port=4
  P_CATH_CNT_SeatHT_W : Outport  Port=5
  wires:
  tSetting_T_User_set_temp_degC/1 -> Calc_Temp_Blowout/1(tSetting_T_User_set_temp_degC)  "tSetting_T_User_set_temp_degC"
  T_ATM_PNT_Outside_degC/1 -> P_PTC_Heater_tgt_calc/1(T_ATM_PNT_Outside_degC), Calc_Temp_Blowout/2(T_ATM_PNT_Outside_degC)  "T_ATM_PNT_Outside_degC"
  T_CABA_PNT_degC/1 -> Calc_Temp_Blowout/3(T_CABA_PNT_T)  "T_CABA_PNT_T"
  Calc_Temp_Blowout/2(T_diff_temp_degC) -> T_SeatHT_Temp_tgt_calc/1(T_diff_temp_degC), P_Heatpomp_Power_tgt_calc/1(T_diff_temp_degC), V_HVAC_Fan_calc/1(T_diff_temp_degC)  "制御用温度差分"
  T_SH_PNT_degC/1 -> T_SeatHT_Temp_tgt_calc/2(T_SH_PNT_degC)  "T_SH_PNT_degC"
  T_AC_PNT_Indoor_degC/1 -> P_Heatpomp_Power_tgt_calc/2(T_AC_PNT_Indoor_degC)  "T_AC_PNT_Indoor_degC"
  T_PTC_PNT_degC/1 -> P_PTC_Heater_tgt_calc/2(T_PTC_PNT_degC)  "T_PTC_PNT_degC"
  V_HVAC_Fan_calc/1(V_CATH_CNT_Aircon_Fan_V) -> V_CATH_CNT_Aircon_Fan_V/1
  P_Heatpomp_Power_tgt_calc/1(P_CATH_CNT_Heatpomp_W) -> P_CATH_CNT_Heatpomp_W/1
  P_PTC_Heater_tgt_calc/1(P_CATH_CNT_PTC_Heater_W) -> P_CATH_CNT_PTC_Heater_W/1
  T_SeatHT_Temp_tgt_calc/1(P_CATH_CNT_SeatHT_W) -> P_CATH_CNT_SeatHT_W/1
  P_Heatpomp_Power_tgt_calc/2(req_V_CATH_CNT_RDFan_V) -> req_V_CATH_CNT_RDFan_V/1
  Calc_Temp_Blowout/1(T_blowout_degC) -> Terminator1/1
  v_VL_PNT_kmph/1 -> Calc_Temp_Blowout/4(v_VL_PNT_kmph)
  Subsystem1/2(Flag_AutoWind) -> P_PTC_Heater_tgt_calc/4(Flag_AutoWind), P_Heatpomp_Power_tgt_calc/4(Flag_AutoWind), V_HVAC_Fan_calc/2(Flag_AutoWind_ON)
  Subsystem1/1(Flag_Aircon) -> P_PTC_Heater_tgt_calc/3(Flag_Aircon), P_Heatpomp_Power_tgt_calc/3(Flag_Aircon)
  tSetting_P_Charger/1 -> Subsystem1/1(tSetting_P_Charger)  "tSetting_P_Charger"

== system EV_thermal_charger_2015a_jmaab/Vehicle/CNT/CHG_CNT/CHG_CNT ==
  note: 0：接続ネゴシエーション
      | 1：初期充電
      | 2：本充電
  note: 本充電開始時間
  note: 初期充電開始時間
  note: 充電信号
      | 充電中は1(=ON)とする
  tSetting_P_Charger : Inport
  V_CHG_PNT_V : Inport  Port=2
  SOC_BT_Hi_PNT_per : Inport  Port=3
  Add : Sum
  Charge_Current_calc : Subsystem
  Compare To Zero : simulink/Logic and Bit Operations/Compare To Zero  relop=>  OutDataTypeStr=boolean
  Constant : Constant  Value=sampling_time
  Constant1 : Constant
  Constant2 : Constant  Value=sampling_time
  Constant3 : Constant  Value=3
  Constant8 : Constant  Value=CHG_CNT_charge_UL_SOC
  Current_rate_limitter : Subsystem
  counter : Subsystem
  counter1 : Subsystem
  tgt_I_CHG_CNT_Charge_A : Outport
  wires:
  tSetting_P_Charger/1 -> Compare To Zero/1  "tSetting_P_Charger"
  Constant/1 -> counter/2(time_step)
  Constant1/1 -> counter/3(count_time)
  Constant2/1 -> counter1/2(time_step)
  Constant3/1 -> counter1/3(count_time)
  counter/1(Out1) -> Add/1
  counter1/1(Out1) -> Add/2
  V_CHG_PNT_V/1 -> Charge_Current_calc/2(V_CHG_PNT_Charge_V)  "V_CHG_PNT_Charge_V"
  SOC_BT_Hi_PNT_per/1 -> Current_rate_limitter/2(SOC_BT_Hi_PNT_per), Charge_Current_calc/3(SOC_BT_Hi_PNT_per)  "SOC_BT_Hi_PNT_per"
  Constant8/1 -> Current_rate_limitter/3(SOC_UL), Charge_Current_calc/4(Maximum_Hi_Batt_SOC)
  Current_rate_limitter/1(tgt_I_CHG_CNT_Charge_A) -> tgt_I_CHG_CNT_Charge_A/1
  Charge_Current_calc/1(Current_tgt) -> Current_rate_limitter/1(Current_tgt_In1)
  Add/1 -> Charge_Current_calc/1(Charge_mode)
  Compare To Zero/1 -> counter1/1(signal), counter/1(signal)

== system EV_thermal_charger_2015a_jmaab/Vehicle/CNT/EL_TH_CNT/ELTH_CNT ==
  T_RDTH_PNT_RDCoolant_degC : Inport
  req_V_CATH_CNT_RDFan_V : Inport  Port=2
  MinMax : MinMax  Function=max  Inputs=2
  RD_Fan_Control : Lookup_n-D  NumberOfTableDimensions=1  BreakpointsForDimension1=ELTH_CNT_V_RDFan_x_T_Coolant  Table=ELTH_CNT_V_RDFan_V  InternalRulePriority=Speed  RndMeth=Simplest  InputSameDT=on
  Waterpomp_Control : Lookup_n-D  NumberOfTableDimensions=1  BreakpointsForDimension1=ELTH_CNT_V_Water_Pump_x_T_Coolant  Table=ELTH_CNT_V_Water_Pump_V  InternalRulePriority=Speed  RndMeth=Simplest  InputSameDT=on
  req_V_ELTH_CNT_RDFan_V : Outport
  V_ELTH_CNT_WP_V : Outport  Port=2
  wires:
  Waterpomp_Control/1 -> V_ELTH_CNT_WP_V/1
  RD_Fan_Control/1 -> MinMax/2
  T_RDTH_PNT_RDCoolant_degC/1 -> Waterpomp_Control/1, RD_Fan_Control/1  "T_RDTH_PNT_RDCoolant_degC"
  req_V_CATH_CNT_RDFan_V/1 -> MinMax/1  "req_V_CATH_CNT_RDFan_V"
  MinMax/1 -> req_V_ELTH_CNT_RDFan_V/1

== system EV_thermal_charger_2015a_jmaab/Vehicle/CNT/MG_CNT/MG_CNT ==
  note: u相の担当トルクは
      | モータートルクの1/3
  tgt_Trq_VCU_CNT_MG_Nm : Inport
  w_MG_PNT_radps : Inport  Port=2
  V_INV_PNT_DC_V : Inport  Port=3
  Constant : Constant  Value=3
  Constant1 : Constant  Value=MG_PNT_eta_MG
  Constant2 : Constant  Value=MG_PNT_MG_Power_factor
  Divide : Product  Inputs=*/
  Divide1 : Product  Inputs=/*
  Divide2 : Product  Inputs=*/
  Memory : Memory
  Memory1 : Memory
  Memory2 : Memory
  Mux : Mux  Inputs=3
  Saturation Dynamic : simulink/Discontinuities/Saturation Dynamic  OutMin=[]  OutMax=[]  OutDataTypeStr=Inherit: Same as second input  OutDataType=fixdt(1, 16)  OutScaling=2^-10  DoSatur=off
  WeakField_Calc : Subsystem
  trq_Gurad_Calc : Subsystem
  インバータ変調率 : Constant  Value=MG_PNT_MG_mod_factor
  Power_factor_MG_CNT : Outport
  tgt_k_MG_CNT_Vpradps : Outport  Port=2
  tgt_I_MG_CNT_UPhase_A : Outport  Port=3
  tag scope: trq_MG_and_Guard=global
  wires:
  V_INV_PNT_DC_V/1 -> Memory/1  "V_INV_PNT_DC_V"
  w_MG_PNT_radps/1 -> Memory2/1  "w_MG_PNT_radps"
  trq_Gurad_Calc/2(LowerLimit) -> Mux/3, Saturation Dynamic/3
  trq_Gurad_Calc/1(UpperLimit) -> Mux/2, Saturation Dynamic/1
  Memory/1 -> WeakField_Calc/4(V_INV_PNT_DC_V)
  Saturation Dynamic/1 -> Divide/1  "U相目標トルク制限後"
  WeakField_Calc/1(k_radps2Volt_tgt) -> Divide1/1, tgt_k_MG_CNT_Vpradps/1
  Memory1/1 -> WeakField_Calc/1(I_MG_tgt)
  Divide2/1 -> Memory1/1, tgt_I_MG_CNT_UPhase_A/1
  Constant/1 -> Divide/2
  Memory2/1 -> trq_Gurad_Calc/1(w_MG_PNT_radps), WeakField_Calc/5(w_MG_PNT_radps)
  tgt_Trq_VCU_CNT_MG_Nm/1 -> Saturation Dynamic/2, Mux/1  "tgt_Trq_VCU_CNT_MG_Nm"
  Divide/1 -> Divide1/2
  Mux/1 -> [trq_MG_and_Guard]  "トルクと制限値"
  Divide1/1 -> Divide2/1
  Constant1/1 -> Divide2/2
  インバータ変調率/1 -> WeakField_Calc/3(MG_Mod_factor)
  Constant2/1 -> Power_factor_MG_CNT/1, WeakField_Calc/2(MG_Power_factor)

== system EV_thermal_charger_2015a_jmaab/Vehicle/CNT/VCU_CNT/VCU_CNT ==
  note: 回生ブレーキ
      | 協調ブレーキ
      | あり
  note: 回生ブレーキ
      | 協調ブレーキ
      | なし
  open_break_Driver_per : Inport
  open_accel_Driver_per : Inport  Port=2
  v_VL_PNT_kmph : Inport  Port=3
  w_MG_PNT_radps : Inport  Port=4
  SOC_BT_Hi_PNT_per : Inport  Port=5
  P_HVAC_PNT_W : Inport  Port=6
  P_DCDC_PNT_W : Inport  Port=7
  Constant : Constant  Value=0
  Constant1 : Constant  Value=VCU_CNT_Cooperative_Control_Brake_flag
  Memory{,1..4} (5 alike) : Memory
  PDfSOC : Subsystem
  ReGenerativeBrake_Calc : Subsystem
  Switch : Switch  Criteria=u2 > Threshold
  trq_MG2_GuardCalc : Subsystem
  trq_MG2_tgtCalc2 : Subsystem
  ユーザ要求駆力算出 : Subsystem
  F_VCU_CNT_re_break_N : Outport
  tgt_Trq_VCU_CNT_MG_Nm : Outport  Port=2
  wires:
  SOC_BT_Hi_PNT_per/1 -> Memory1/1  "SOC_BT_Hi_PNT_per"
  open_accel_Driver_per/1 -> ユーザ要求駆力算出/1(open_accel_Driver_per)  "open_accel_Driver_per"
  v_VL_PNT_kmph/1 -> Memory/1
  ユーザ要求駆力算出/1(P_vehicle_tgt) -> trq_MG2_tgtCalc2/1(User_Power_req)
  PDfSOC/2(PSoFout) -> trq_MG2_GuardCalc/3(PSoFout)
  PDfSOC/1(PSoFin) -> trq_MG2_GuardCalc/2(PSoFin)
  w_MG_PNT_radps/1 -> Memory3/1  "w_MG_PNT_radps"
  open_break_Driver_per/1 -> ユーザ要求駆力算出/2(open_break_Driver_per), ReGenerativeBrake_Calc/2(open_break_Driver_per)  "open_break_Driver_per"
  Switch/1 -> trq_MG2_tgtCalc2/6(trq_R_brake_tgt)
  P_HVAC_PNT_W/1 -> Memory4/1  "P_HVAC_PNT_W"
  ユーザ要求駆力算出/2(trq_motor_UserAcc_tgt) -> trq_MG2_tgtCalc2/3(trq_motor_UserAcc_tgt)
  trq_MG2_GuardCalc/1(trq_MG2_UpperGuard) -> trq_MG2_tgtCalc2/4(trq_MG2_UpperGuard)
  trq_MG2_GuardCalc/2(trq_MG2_LowerGuard) -> trq_MG2_tgtCalc2/5(trq_MG2_LowerGuard)
  Memory/1 -> ユーザ要求駆力算出/3(v_VL_PNT_kmph), ReGenerativeBrake_Calc/1(v_VL_PNT_kmph)  "v_VL_PNT_kmph"
  Memory1/1 -> PDfSOC/1(SOC_BT_Hi_PNT_per)
  Memory3/1 -> trq_MG2_GuardCalc/1(w_MG_PNT_radps), trq_MG2_tgtCalc2/2(w_MG_PNT_radps)
  trq_MG2_tgtCalc2/2(F_VCU_CNT_re_break_N) -> F_VCU_CNT_re_break_N/1
  Memory4/1 -> trq_MG2_GuardCalc/4(P_HVAC_PNT_W)
  trq_MG2_tgtCalc2/1(tgt_Trq_VCU_CNT_MG_Nm) -> tgt_Trq_VCU_CNT_MG_Nm/1
  P_DCDC_PNT_W/1 -> Memory2/1  "P_DCDC_PNT_W"
  Memory2/1 -> trq_MG2_GuardCalc/5(P_DCDC_PNT_W)
  Constant1/1 -> Switch/2
  Constant/1 -> Switch/3
  ReGenerativeBrake_Calc/1(trq_R_brake_tgt) -> Switch/1

== system EV_thermal_charger_2015a_jmaab/Vehicle/DCDC_PNT/DCDC_PNT/Controller ==
  note: 0割防止
  Target V : Inport
  V : Inport  Port=2
  Constant : Constant  Value=0.01
  Divide : Product  Inputs=*/
  MinMax : MinMax  Function=max  Inputs=2
  Gain : Outport
  wires:
  Divide/1 -> Gain/1
  Target V/1 -> Divide/1
  MinMax/1 -> Divide/2
  V/1 -> MinMax/1
  Constant/1 -> MinMax/2

== system EV_thermal_charger_2015a_jmaab/Vehicle/DCDC_PNT/DCDC_PNT/resi1 ==
  In1 : Inport
  Constant1 : Constant  Value=DCDC_PNT_R_conv_lo
  Product4 : Product  Inputs=*/  RndMeth=Zero
  Out1 : Outport
  wires:
  In1/1 -> Product4/1
  Constant1/1 -> Product4/2
  Product4/1 -> Out1/1

== system EV_thermal_charger_2015a_jmaab/Vehicle/DTTH/DTTH_PNT/DFTH_PNT ==
  note: T/Mブロックへの熱量
  note: DFオイルの
      | 熱容量
  note: DFブロックの
      | 熱容量
  Temp_ini : Inport
  "T_ATM_PNT_DF_K " : Inport  Port=2
  PHI_DF_PNT_W : Inport  Port=3
  "T_TMTH_PNT_DFTH_K " : Inport  Port=4
  DFBlock2Air_Heat_Resistance : Subsystem
  DFBlock_Heat_Capacity : Subsystem
  DFOil2DFBlock_Heat_Resistance : Subsystem
  DFOil_Heat_Capacity : Subsystem
  K->degC1 : Subsystem
  TMBlock2DFBlock_Heat_Resistance : Subsystem
  "PHI_DFTH_PNT_ATM_W " : Outport
  T_DFTH_PNT_TM_K : Outport  Port=2
  "PHI_DFTH_PNT_TMTH_W " : Outport  Port=3
  tag scope: tScope_T_DFBlock_degC=global
  wires:
  DFOil_Heat_Capacity/2(T_DFOil2_K) -> DFOil2DFBlock_Heat_Resistance/2("T_DFOil_Resi2_K ")
  DFOil2DFBlock_Heat_Resistance/2(PHI_DFOil_Resi2_W) -> DFOil_Heat_Capacity/3("PHI_DFOil2_W ")
  DFOil2DFBlock_Heat_Resistance/1(PHI_DFBlock_Resi1_W) -> DFBlock_Heat_Capacity/2("PHI_DFBlock1_W ")
  DFBlock2Air_Heat_Resistance/2("PHI_DFBlock_Resi3_W ") -> DFBlock_Heat_Capacity/4(PHI_DFBlock3_W)
  DFBlock2Air_Heat_Resistance/1("PHI_DF_Air_Resi1_W ") -> "PHI_DFTH_PNT_ATM_W "/1  "PHI_DFTH_PNT_ATM_W"
  TMBlock2DFBlock_Heat_Resistance/1("PHI_DFBlock_Resi2_W ") -> DFBlock_Heat_Capacity/3("PHI_DFBlock2_W ")
  DFBlock_Heat_Capacity/2(T_DFBlock2_K) -> TMBlock2DFBlock_Heat_Resistance/1("T_DFBlock_Resi2_K ")
  "T_TMTH_PNT_DFTH_K "/1 -> TMBlock2DFBlock_Heat_Resistance/2("T_TMBlock_Resi4_K ")
  TMBlock2DFBlock_Heat_Resistance/2("PHI_TMBlock_Resi4_W ") -> "PHI_DFTH_PNT_TMTH_W "/1
  PHI_DF_PNT_W/1 -> DFOil_Heat_Capacity/2(PHI_DFOil1_W)
  Temp_ini/1 -> DFBlock_Heat_Capacity/1(Temp_ini), DFOil_Heat_Capacity/1(Temp_ini)
  K->degC1/1(degC) -> [tScope_T_DFBlock_degC]
  "T_ATM_PNT_DF_K "/1 -> DFBlock2Air_Heat_Resistance/2(T_DF_Air_Resi1_K)
  DFBlock_Heat_Capacity/3("T_DFBlock3_K ") -> DFBlock2Air_Heat_Resistance/1("T_DFBlock_Resi3_K "), K->degC1/1(K)
  DFBlock_Heat_Capacity/1("T_DFBlock1_K ") -> DFOil2DFBlock_Heat_Resistance/1(T_DFBlock_Resi1_K)
  DFOil_Heat_Capacity/1("T_DFOil1_K ") -> T_DFTH_PNT_TM_K/1  "T_DFTH_PNT_TM_K"

== system EV_thermal_charger_2015a_jmaab/Vehicle/DTTH/DTTH_PNT/K->degC6 ==
  K : Inport
  Constant2 : Constant  Value=K2degC
  Sum : Sum  Inputs=++|
  degC : Outport
  wires:
  K/1 -> Sum/2
  Constant2/1 -> Sum/1
  Sum/1 -> degC/1

== system EV_thermal_charger_2015a_jmaab/Vehicle/DTTH/DTTH_PNT/TMTH_PNT ==
  note: TFの
      | 熱容量
  note: T/Mブロックの
      | 熱容量
  note: DFブロックからの熱量
  note: TMからの熱量
  note: T/Mブロックから大気へ
      | 放熱する熱量
  note: モーターハウジングからの熱量
  Temp_ini : Inport
  PHI_TM_PNT_W : Inport  Port=2
  "PHI_MGTH_PNT_PTTH_W " : Inport  Port=3
  "T_ATM_PNT_TM_K " : Inport  Port=4
  "PHI_DFTH_PNT_TMTH_W " : Inport  Port=5
  K->degC1 : Subsystem
  TF2TMBlock_Heat_Resistance : Subsystem
  TF_Heat_Capacity : Subsystem
  TMBlock2Air_Heat_Resistance : Subsystem
  TMBlock_Heat_Capacity : Subsystem
  T_TMTH_PNT_DFTH_K : Outport
  PHI_TMTH_PNT_ATM_W : Outport  Port=2
  T_TMTH_PNT_ELTH_K : Outport  Port=3
  "T_TMTH_PNT_TM_K " : Outport  Port=4
  T_TF_K : Outport  Port=5
  tag scope: tScope_T_TMBlock_degC=global
  wires:
  TF_Heat_Capacity/2(T_TF2_K) -> TF2TMBlock_Heat_Resistance/2("T_TF_Resi2_K ")
  TF2TMBlock_Heat_Resistance/2(PHI_TF_Resi2_W) -> TF_Heat_Capacity/3(PHI_TF2_W)
  TMBlock_Heat_Capacity/1(T_TMBlock1_K) -> TF2TMBlock_Heat_Resistance/1("T_TMBlock_Resi1_K ")
  TF2TMBlock_Heat_Resistance/1(PHI_TMBlock_Resi1_W) -> TMBlock_Heat_Capacity/2(PHI_TMBlock1_W)
  TF_Heat_Capacity/1(T_TF1_K) -> T_TF_K/1, "T_TMTH_PNT_TM_K "/1  "T_TMTH_PNT_TM_K"
  TMBlock2Air_Heat_Resistance/2(PHI_TMBlock_Resi3_W) -> TMBlock_Heat_Capacity/3(PHI_TMBlock2_W)
  TMBlock_Heat_Capacity/2(T_TMBlock2_K) -> TMBlock2Air_Heat_Resistance/2("T_TMBlock_Resi3_K ")
  TMBlock_Heat_Capacity/3(T_TMBlock3_K) -> T_TMTH_PNT_DFTH_K/1  "T_TMTH_PNT_DFTH_K"
  "PHI_DFTH_PNT_TMTH_W "/1 -> TMBlock_Heat_Capacity/4(PHI_TMBlock3_W)
  "T_ATM_PNT_TM_K "/1 -> TMBlock2Air_Heat_Resistance/1(T_TM_Air_Resi1_K)
  TMBlock2Air_Heat_Resistance/1("PHI_TM_Air_Resi1_W ") -> PHI_TMTH_PNT_ATM_W/1  "PHI_TMTH_PNT_ATM_W"
  TMBlock_Heat_Capacity/4(T_TMBlock4_K) -> K->degC1/1(K), T_TMTH_PNT_ELTH_K/1  "T_TMTH_PNT_ELTH_K"
  Temp_ini/1 -> TMBlock_Heat_Capacity/1(Temp_ini), TF_Heat_Capacity/1(Temp_ini)
  K->degC1/1(degC) -> [tScope_T_TMBlock_degC]
  "PHI_MGTH_PNT_PTTH_W "/1 -> TMBlock_Heat_Capacity/5(PHI_TMBlock4_W)
  PHI_TM_PNT_W/1 -> TF_Heat_Capacity/2(PHI_TF1_W)

== system EV_thermal_charger_2015a_jmaab/Vehicle/DT_PNT/DF_PNT/DriveShaft ==
  "w_DF_PNT_radps " : Inport
  "w_TR_PNT_radps " : Inport  Port=2
  Add : Sum  Inputs=+-
  Add1 : Sum
  Discrete-Time Integrator : DiscreteIntegrator  InitialConditionSetting=State (most efficient)  SampleTime=sampling_time  LowerSaturationLimit=0  ICPrevOutput=DiscIntNeverNeededParam  ICPrevScaledInput=DiscIntNeverNeededParam
  Gain : Gain  Gain=-1
  Gain1 : Gain  Gain=DF_PNT_Driveshaft_spring
  Gain2 : Gain  Gain=DF_PNT_Driveshaft_damper
  "Trq_DF_PNT_Nm " : Outport
  Trq_DF_PNT_DN_Nm : Outport  Port=2
  wires:
  Discrete-Time Integrator/1 -> Gain1/1
  "w_DF_PNT_radps "/1 -> Add/1
  "w_TR_PNT_radps "/1 -> Add/2
  Gain1/1 -> Add1/1
  Gain2/1 -> Add1/2
  Gain/1 -> "Trq_DF_PNT_Nm "/1
  Add/1 -> Discrete-Time Integrator/1, Gain2/1
  Add1/1 -> Trq_DF_PNT_DN_Nm/1, Gain/1

== system EV_thermal_charger_2015a_jmaab/Vehicle/DT_PNT/TM_PNT/Flywheel1 ==
  Trq_DF_PNT_UP_Nm : Inport
  Trq_TM_Flywheel_UP : Inport  Port=2
  Discrete-Time Integrator : DiscreteIntegrator  InitialConditionSetting=State (most efficient)  SampleTime=sampling_time  LowerSaturationLimit=0  ICPrevOutput=DiscIntNeverNeededParam  ICPrevScaledInput=DiscIntNeverNeededParam
  Divide : Product  Inputs=/*
  Inertia : Constant  Value=TM_PNT_TM_Inertia
  Sum : Sum  Inputs=++|
  w_TM_PNT_DN_radps : Outport
  "w_ROT_TM_Flywheel_UP " : Outport  Port=2
  wires:
  Trq_DF_PNT_UP_Nm/1 -> Sum/1
  Sum/1 -> Divide/2
  Inertia/1 -> Divide/1
  Divide/1 -> Discrete-Time Integrator/1
  Discrete-Time Integrator/1 -> w_TM_PNT_DN_radps/1, "w_ROT_TM_Flywheel_UP "/1
  Trq_TM_Flywheel_UP/1 -> Sum/2

== system EV_thermal_charger_2015a_jmaab/Vehicle/ELTH/ELTH_PNT/INVTH_PNT ==
  note: モーターハウジングへの熱量
  note: ヒートシンクの
      | 熱容量
  note: インバータ筐体の
      | 熱容量
  note: 冷却水からの熱量
  Temp_ini : Inport
  PHI_INV_PNT_W : Inport  Port=2
  T_ATM_PNT_INV_K : Inport  Port=3
  T_MGTH_PNT_INVTH_K : Inport  Port=4
  PHI_RD_PNT_INVTH_W : Inport  Port=5
  INVBlock2Air_Heat_Resistance : Subsystem
  INVBlock_Heat_Capacity : Subsystem
  INVHeatsink2INVBlock_Heat_Resistance : Subsystem
  INVTH_Heatsink_Heat_Capacity : Subsystem
  K->degC1 : Subsystem
  K->degC2 : Subsystem
  MG2INVBlock_Heat_Resistance : Subsystem
  T_INVHeatsink_K : Outport
  T_INVTH_PNT_K : Outport  Port=2
  PHI_INVTH_PNT_ATM_W : Outport  Port=3
  T_INVTH_PNT_RD_K : Outport  Port=4
  PHI_INVTH_PNT_MGTH_W : Outport  Port=5
  tag scope: tScope_T_INVBlock_degC=global, tScope_T_INVHeatsink_degC=global
  wires:
  INVBlock_Heat_Capacity/3(T_INVBlock1_K) -> INVHeatsink2INVBlock_Heat_Resistance/2(T_INVBlock_Resi1_K)
  INVHeatsink2INVBlock_Heat_Resistance/1(PHI_INVBlock_Resi1_W) -> INVBlock_Heat_Capacity/3(PHI_INVBlock1_W)
  INVBlock2Air_Heat_Resistance/2(PHI_INVBlock_Resi3_W) -> INVBlock_Heat_Capacity/4(PHI_INVBlock3_W)
  INVBlock_Heat_Capacity/2(T_INVBlock3_K) -> INVBlock2Air_Heat_Resistance/2(T_INVBlock_Resi3_K), K->degC1/1(K)
  INVBlock2Air_Heat_Resistance/1(PHI_INV2Air_Resi1_W) -> PHI_INVTH_PNT_ATM_W/1  "PHI_INVTH_PNT_ATM_W"
  MG2INVBlock_Heat_Resistance/1(PHI_INVBlock_Resi2_W) -> INVBlock_Heat_Capacity/1(PHI_INVBlock2_W)
  INVBlock_Heat_Capacity/1(T_INVBlock2_K) -> MG2INVBlock_Heat_Resistance/1(T_INVBlock_Resi2_K)
  T_MGTH_PNT_INVTH_K/1 -> MG2INVBlock_Heat_Resistance/2(T_MGBlock_Resi4_K)
  MG2INVBlock_Heat_Resistance/2(PHI_MGBlock_Resi4_W) -> PHI_INVTH_PNT_MGTH_W/1  "HI_INVTH_PNT_MGTH_W"
  INVTH_Heatsink_Heat_Capacity/1(T_INVTH_Heatsink1_K) -> T_INVTH_PNT_K/1  "T_INVTH_PNT_K"
  PHI_INV_PNT_W/1 -> INVTH_Heatsink_Heat_Capacity/2(PHI_INVTH_Heatsink1_W)
  T_ATM_PNT_INV_K/1 -> INVBlock2Air_Heat_Resistance/1(T_INV2Air_Resi1_K)
  INVTH_Heatsink_Heat_Capacity/3(T_INVTH_Heatsink3_K) -> T_INVTH_PNT_RD_K/1, K->degC2/1(K), T_INVHeatsink_K/1  "T_INVHeatsink_K"
  PHI_RD_PNT_INVTH_W/1 -> INVTH_Heatsink_Heat_Capacity/3(PHI_INVTH_Heatsink3_W)
  INVTH_Heatsink_Heat_Capacity/2(T_INVTH_Heatsink2_K) -> INVHeatsink2INVBlock_Heat_Resistance/1(T_INVHeatsink_Resi2_K)
  INVHeatsink2INVBlock_Heat_Resistance/2(PHI_INVHeatsink_Resi2_W) -> INVTH_Heatsink_Heat_Capacity/4(PHI_INVTH_Heatsink2_W)
  Temp_ini/1 -> INVTH_Heatsink_Heat_Capacity/1(Temp_ini), INVBlock_Heat_Capacity/2(Temp_ini)
  K->degC2/1(degC) -> [tScope_T_INVHeatsink_degC]
  K->degC1/1(degC) -> [tScope_T_INVBlock_degC]

== system EV_thermal_charger_2015a_jmaab/Vehicle/ELTH/ELTH_PNT/K->degC1 ==
  K : Inport
  Constant2 : Constant  Value=K2degC
  Sum : Sum  Inputs=++|
  degC : Outport
  wires:
  K/1 -> Sum/2
  Constant2/1 -> Sum/1
  Sum/1 -> degC/1
